simulink subsystem "acc_cbf_test"  (R2025b)
settings: Solver=VariableStepAuto  StartTime=0.0  StopTime=10.0  RelTol=1e-3
settings Model: Creator=sanborkl  LastModifiedBy=sanborkl

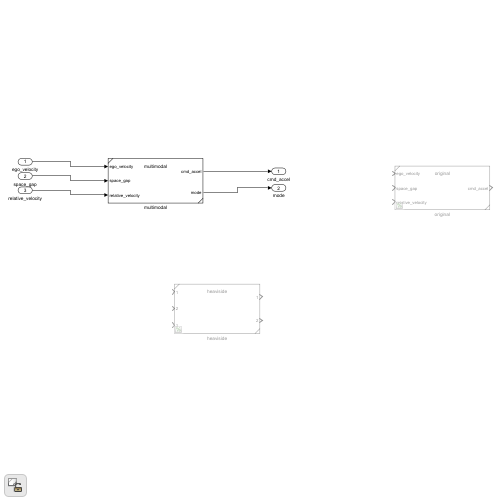
[thumbnail: Simulink's stored preview of the top-level diagram]
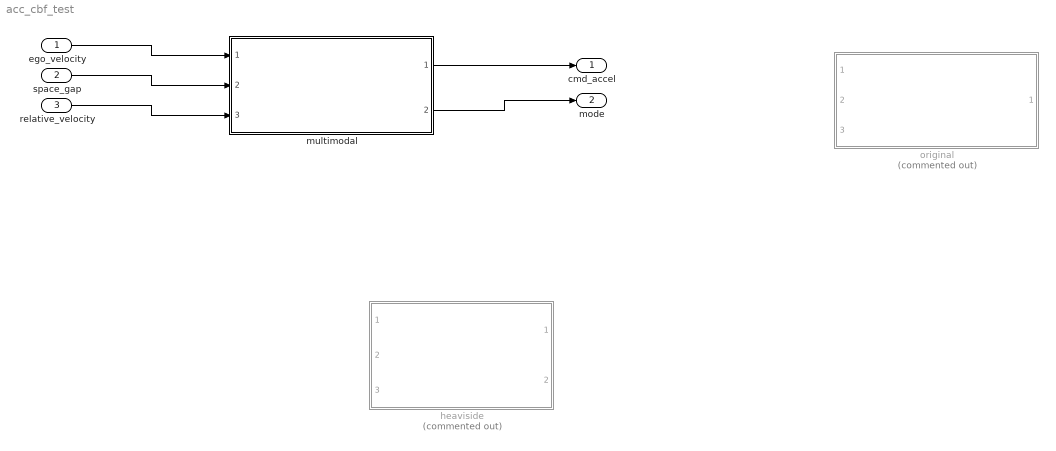
== system acc_cbf_test ==
  ego_velocity : Inport
  space_gap : Inport  Port=2
  relative_velocity : Inport  Port=3
  heaviside : Subsystem  Commented=on  ReferencedSubsystem=heaviside
  multimodal : Subsystem  ReferencedSubsystem=multimodal
  original : Subsystem  Commented=on  ReferencedSubsystem=original
  cmd_accel : Outport
  mode : Outport  Port=2
  wires:
  multimodal/1 -> cmd_accel/1
  multimodal/2 -> mode/1
  ego_velocity/1 -> multimodal/1
  space_gap/1 -> multimodal/2
  relative_velocity/1 -> multimodal/3
